simulink model "sfunc_level2"  (R2021a)
settings: Solver=FixedStepDiscrete  StartTime=0.0  StopTime=10.0  RelTol=1e-3
PreLoadFcn:
  | Simulink.importExternalCTypes('./C_Files/ex_myTypes_LCT.h');
  | clear ans
CloseFcn:
  | clear all
  | try
  | rmdir slprj\ s
  | catch
  | end
  | try
  | folder_name = [bdroot '*'];
  | rmdir(folder_name,'s')
  | catch
  | end
  | try
  | file_temp_name = [bdroot '.slxc'];
  | delete(file_temp_name)
  | %%delete *.mexw64
  | catch
  | end
  | clear folder_name file_temp_name
settings Model: Creator=jetson  LastModifiedBy=jetson
settings DataIOCC: SaveOutput=off  SignalLogging=off  DSMLogging=off  SaveTime=off  ReturnWorkspaceOutputs=off
settings OptimizationCC: DefaultParameterBehavior=Inlined  EnhancedBackFolding=on  PassReuseOutputArgsAs=Individual arguments  ZeroExternalMemoryAtStartup=off  ZeroInternalMemoryAtStartup=off  OptimizeBlockOrder=speed  DifferentSizesBufferReuse=on  OptimizationCustomize=off  EfficientTunableParamExpr=on
settings DebuggingCC: ParameterTunabilityLossMsg=error
settings SFSimCC: MATLABDynamicMemAlloc=off
settings RTWCC: SystemTargetFile=ert.tlc  GenCodeOnly=on  TemplateMakefile=ert_default_tmf  GenerateReport=on  CustomSource=ex_mySrc_LCT.c  IncludeHyperlinkInReport=on  LaunchReport=on  GenerateTraceInfo=on
settings CodeAppCC: ForceParamTrailComments=on  IgnoreCustomStorageClasses=off  OperatorAnnotations=on  SimulinkDataObjDesc=on  SFDataObjDesc=on  InsertBlockDesc=on
settings ERTTargetCC: TargetLangStandard=C99 (ISO)  GenerateSampleERTMain=on  InlinedParameterPlacement=NonHierarchical  ERTCustomFileTemplate=example_file_process.tlc

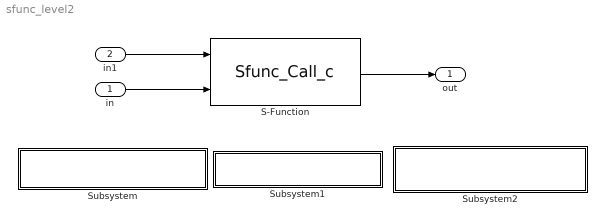
== system sfunc_level2 ==
  in : Inport  ClipboardFcn=Data Type : %<OutDataTypeStr>  OutDataTypeStr=Bus: sigStructType
      settings: AttributesFormatString=Data Type : %<OutDataTypeStr>
  in1 : Inport  ClipboardFcn=Data Type : %<OutDataTypeStr>  Port=2  OutDataTypeStr=Bus: paramStructType
      settings: AttributesFormatString=Data Type : %<OutDataTypeStr>
  S-Function : S-Function  FunctionName=Sfunc_Call_c  SFunctionDeploymentMode=off  EnableBusSupport=off
  Subsystem : Subsystem
      settings: OpenFcn=mex -IC_Files ./Sfunction_TLC/Sfunc_Call_c.c ./C_Files/ex_mySrc_LCT.c -outdir ./Sfunction_TLC/
      mask Display:
      | color('r')
      | disp('double click will compile Sfunc_Call_c.c')
  Subsystem1 : Subsystem
      settings: OpenFcn=Sfunc_Call_c ex_mySrc_LCT.c
      mask Display:
      | color('r')
      | disp('double click will open Sfunc_Call_c.c')
  Subsystem2 : Subsystem
      settings: OpenFcn=edit Sfunc_Call_c.tlc
      mask Display:
      | color('r')
      | disp('double click will compile Sfunc_Call_c.tlc')
  out : Outport  OutDataTypeStr=Bus: sigStructType
      settings: AttributesFormatString=Data Type : %<OutDataTypeStr>
  wires:
  S-Function/1 -> out/1
  in1/1 -> S-Function/1
  in/1 -> S-Function/2

== system sfunc_level2/Subsystem ==

== system sfunc_level2/Subsystem1 ==

== system sfunc_level2/Subsystem2 ==
